simulink model "PruebaSensores"  (R2023b)
settings: Solver=VariableStepAuto  StartTime=0.0  StopTime=10.0  RelTol=1e-3
libraries: arduinolib x2
settings Model: Creator=Diego  LastModifiedBy=Usuario_UMA

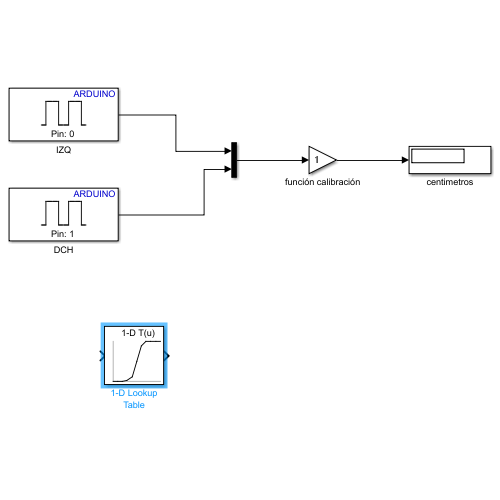
[thumbnail: Simulink's stored preview of the top-level diagram]
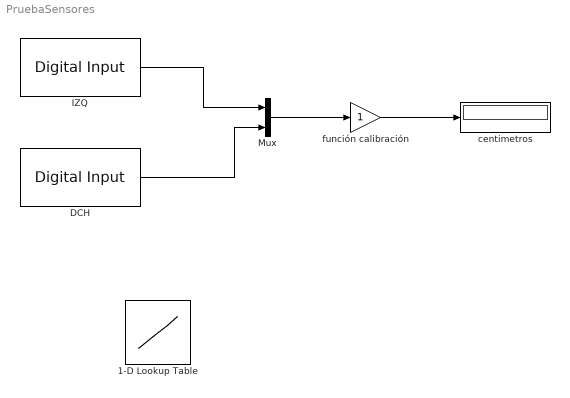
== system PruebaSensores ==
  1-D Lookup Table : Lookup_n-D  NumberOfTableDimensions=1  BreakpointsForDimension1=[-5:5]  Table=tanh([-5:5])  InternalRulePriority=Speed  RndMeth=Simplest
  DCH : arduinolib/Digital Input  pinNumber=1  mode=Default  Direction=input  SampleTime=0.1  blockPlatform=arduino
  IZQ : arduinolib/Digital Input  pinNumber=0  mode=Default  Direction=input  SampleTime=0.1  blockPlatform=arduino
  Mux : Mux  Inputs=2
  centimetros : Display
  función calibración : Gain
  wires:
  IZQ/1 -> Mux/1
  DCH/1 -> Mux/2
  Mux/1 -> función calibración/1
  función calibración/1 -> centimetros/1
